simulink model "lab02_class"  (R2018a)
settings: Solver=VariableStepAuto  StartTime=0.0  StopTime=tf  MaxStep=maxstep  RelTol=tol  AbsTol=tol
values from neighbouring files (symbols this model uses):
  b = 1    [Lab2_script_class.m]
  f = 10    [Lab2_script_class.m]
  m = 100    [Lab2_script_class.m]
  v0 = 0    [Lab2_script_class.m]
settings Model: Creator=rodrigue  LastModifiedBy=rodrigue

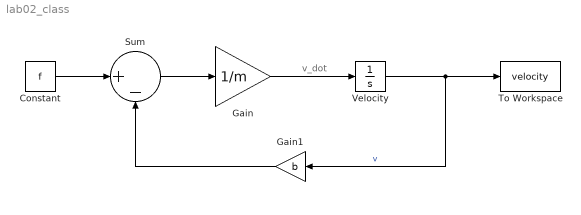
== system lab02_class ==
  note: v_dot
  Constant : Constant  Value=f
  Gain : Gain  Gain=1/m
  Gain1 : Gain  Gain=b
  Sum : Sum  Inputs=|+-
  To Workspace : ToWorkspace  VariableName=velocity  SampleTime=-1
  Velocity : Integrator  InitialCondition=v0
  wires:
  Sum/1 -> Gain/1
  Gain/1 -> Velocity/1
  Velocity/1 -> To Workspace/1, Gain1/1  "v"
  Gain1/1 -> Sum/2
  Constant/1 -> Sum/1
